simulink model "Traverse_system"  (R2022b)
settings: Solver=VariableStepAuto  StartTime=0.0  StopTime=30  RelTol=1e-3
undefined symbols (not defined in the file): C_pi_pod_trav_Ki, C_pi_pod_trav_Kp, C_pi_trav_gyro_simple, C_pi_trav_techo, gain_pod_trav, k_feed_gun_trav, k_feed_pod_trav, k_tgun_inv_plant, k_tpod_inv_plant, linear_feed_forward_GUN_trav_dist, linear_feed_forward_POD_trav_dist, linear_tgun_inv_plant, linear_tpod_inv_plant, trav_gyro_gain, trav_gyro_notch, trav_tacho_notch, trav_techo_plent_gain
libraries: slpidlib x4, simulink x1
settings Model: PacingRate=0.001000  Creator=ohadformanair  LastModifiedBy=ohadformanair
settings SolverCC: ZeroCrossAlgorithm=Adaptive
settings DataIOCC: SaveFormat=StructureWithTime
settings OptimizationCC: BlockReduction=off  OptimizeBlockIOStorage=off  BufferReuse=off
settings DebuggingCC: MaskedZcDiagnostic=none  IgnoredZcDiagnostic=none
settings ModelReferenceCC: EnableRefExpFcnMdlSchedulingChecks=on

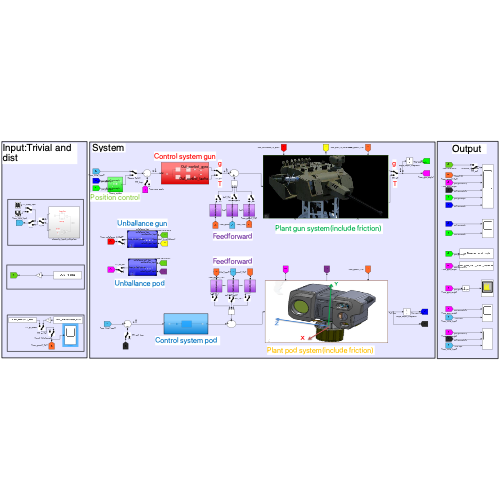
[thumbnail: Simulink's stored preview of the top-level diagram]
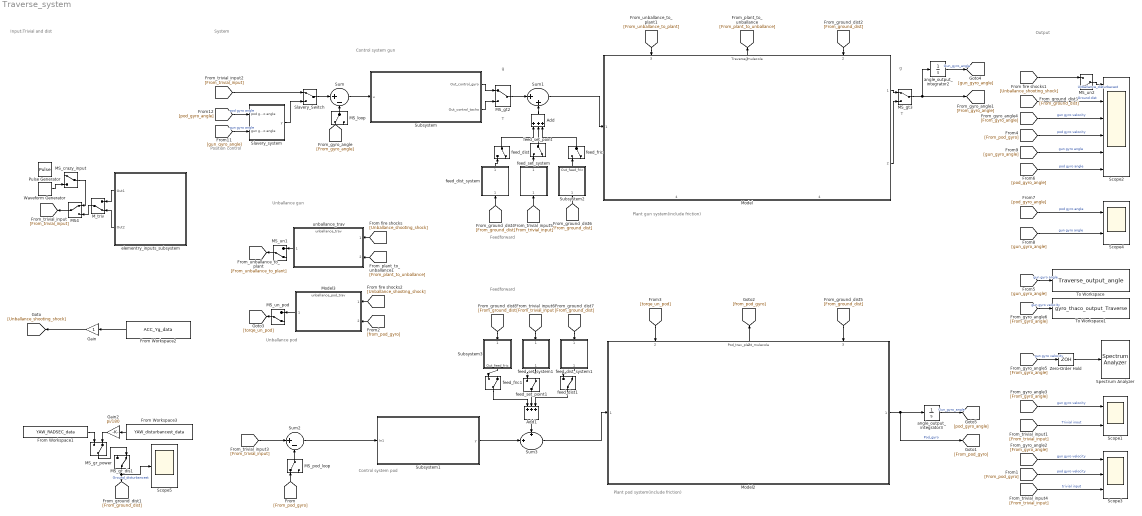
== system Traverse_system ==
  note: g
  note: g
  note: T
  note: T
  note: Plant gun system(include friction)
  note: Control system gun
  note: Unballance gun
  note: Input:Trivial and dist
  note: System
  note: Output
  note: Feedforward
  note: Plant pod system(include friction)
  note: Control system pod
  note: Unballance pod
  note: Position control
  note: Feedforward
  Add : Sum  Inputs=+++
  Add1 : Sum  Inputs=+++
  From Workspace1 : FromWorkspace  VariableName=YAW_RADSEC_data  SampleTime=-1
  From Workspace2 : FromWorkspace  VariableName=ACC_Yg_data  SampleTime=-1
  From Workspace3 : FromWorkspace  VariableName=YAW_disturbancest_data  SampleTime=-1
  Gain : Gain
  Gain2 : Gain  Gain=pi/180
  MS4 : ManualSwitch
  MS_crazy_input : ManualSwitch
  MS_gr_dis1 : ManualSwitch  CurrentSetting=0
  MS_gr_power : ManualSwitch  CurrentSetting=0
  MS_gt2 : ManualSwitch
  MS_gt3 : ManualSwitch
  MS_loop : ManualSwitch
  MS_pod_loop : ManualSwitch
  MS_un1 : ManualSwitch  CurrentSetting=0
  MS_un2 : ManualSwitch  CurrentSetting=0
  MS_un_pod : ManualSwitch  CurrentSetting=0
  M_triv : ManualSwitch  CurrentSetting=0
  Model : ModelReference  ModelNameDialog=Traverse_mulecola.slx  SimulationMode=Normal  ModelReferenceVersion=2.15
      settings: PortSchema="{\"entries\":[{\"content\":{\"sides\":[{\"content\":{\"connectorIds\":[\"In1\"]},\"type\":\"ConnectorPlacement.EquallySpacedRectSide\",\"uuid\":\"eac8caca-da38-417c-b045-6ec85fbd043e\"},{\"content\":{\"connectorIds\":[\"Out1\",\"Out2\"],\"side\":\"RIGHT\"},\"type\":\"ConnectorPlacement.EquallySpacedRectSide\",\"uuid\":\"64e84338-5cc1-4477-948e-9d784403bbd8\"},{\"content\":{\"connectorIds\":[\"In3\",\"Out3\",\"In2\"],\"side\":\"TOP\"},\"type\":\"ConnectorPlacement.EquallySpacedRectSide\",\"uuid\":\"1763b0b1-bf18-4a22-9773-91c6e4565572\"},{\"content\":{\"connectorIds\":[\"Out4\",\"In4\"],\"side\":\"BOTTOM\"},\"type\":\"ConnectorPlacement.EquallySpacedRectSide\",\"uuid\":\"ba992d88-ce65-42ad-a7d1-2242850eefcb\"}]},\"type\":\"ConnectorPlacement.EquallySpacedConnector\",\"uuid\":\"eba2f321-7b3d-4eb1-ab17-9114bc836124\"}],\"packageUris\":[\"http://schema.mathworks.com/mf0/Connector/R2020b\"],\"version\":\"1.0\"}"
      mask Display: image('/Users/ohadformanair/Desktop/צילום מסך 2022-12-07 ב-4.16.46.png'); % Use "Edit Image" on toolstrip to change.
  Model2 : ModelReference  ModelNameDialog=Pod_trav_plant_mulecola  SimulationMode=Normal  ModelReferenceVersion=1.15
      settings: PortSchema="{\"entries\":[{\"content\":{\"sides\":[{\"content\":{\"connectorIds\":[\"In1\"]},\"type\":\"ConnectorPlacement.EquallySpacedRectSide\",\"uuid\":\"257dd348-bb73-4a25-bb22-0aa44bc5c6b9\"},{\"content\":{\"connectorIds\":[\"Out1\"],\"side\":\"RIGHT\"},\"type\":\"ConnectorPlacement.EquallySpacedRectSide\",\"uuid\":\"83205adf-7330-4a40-93ca-0cec5d3c6531\"},{\"content\":{\"connectorIds\":[\"In2\",\"Out2\",\"In3\"],\"side\":\"TOP\"},\"type\":\"ConnectorPlacement.EquallySpacedRectSide\",\"uuid\":\"cb3612bd-e216-4a60-bf79-1bea0ce7796e\"}]},\"type\":\"ConnectorPlacement.EquallySpacedConnector\",\"uuid\":\"f84f5dbe-ed6b-457b-b8fc-4d1969f08882\"}],\"packageUris\":[\"http://schema.mathworks.com/mf0/Connector/R2020b\"],\"version\":\"1.0\"}"
      mask Display: image('/Users/ohadformanair/Desktop/צילום מסך 2022-12-07 ב-4.14.47.png'); % Use "Edit Image" on toolstrip to change.
  Model3 : ModelReference  ModelNameDialog=unballance_pod_trav.slx  SimulationMode=Normal  ModelReferenceVersion=1.12
  Pulse Generator : DiscretePulseGenerator  PulseType=Time based  Period=1  PulseWidth=50
  Scope1 : Scope  NumInputPorts=2
  Scope2 : Scope  NumInputPorts=6
  Scope3 : Scope  NumInputPorts=3
  Scope4 : Scope  NumInputPorts=2
  Scope5 : Scope
  Slavery_Switch : ManualSwitch
  Slavery_system : Subsystem
  Spectrum Analyzer : SpectrumAnalyzer
  Subsystem : Subsystem
  Subsystem1 : Subsystem  TreatAsAtomicUnit=on
  Subsystem2 : Subsystem
  Subsystem3 : Subsystem
  Sum : Sum  Inputs=|+-
  Sum1 : Sum  Inputs=|++
  Sum2 : Sum  Inputs=|+-
  Sum3 : Sum  Inputs=+|+||
  To Workspace : ToWorkspace  VariableName=Traverse_output_angle  SaveFormat=Timeseries  SampleTime=-1
  To Workspace1 : ToWorkspace  VariableName=gyro_thaco_output_Traverse  SaveFormat=Timeseries  SampleTime=-1
  Waveform Generator : simulink/Sources/Waveform Generator  OutMin=[]  OutMax=[]  OutDataTypeStr=double  SelectedSignal=1  Signals=sin(sawtooth(1,2,0),1,2)+Square(1,2,0,50)#Square(1,2,0,50)  BlockNames=MultiportSwitch_bb3116ca3c8c4cb#MultiportSwitch_6d83ebdfd0d2480  SampleTime=0.01
  Zero-Order Hold : ZeroOrderHold  SampleTime=0.001
  angle_output_integrator2 : Integrator
  angle_output_integrator3 : Integrator
  elementry_inputs_subsystem : Subsystem
  feed_dist : ManualSwitch  CurrentSetting=0
  feed_dist1 : ManualSwitch  CurrentSetting=0
  feed_dist_system : Subsystem
  feed_dist_system1 : Subsystem
  feed_fric : ManualSwitch  CurrentSetting=0
  feed_fric1 : ManualSwitch  CurrentSetting=0
  feed_set_point : ManualSwitch  CurrentSetting=0
  feed_set_point1 : ManualSwitch  CurrentSetting=0
  feed_set_system : Subsystem
  feed_set_system1 : Subsystem
  unballance_trav : ModelReference  ModelNameDialog=unballance_trav.slx  SimulationMode=Normal  ModelReferenceVersion=1.14
  wires:
  MS_loop/1 -> Sum/2
  MS_gt3/1 -> angle_output_integrator2/1, [From_gyro_angle]
  Model/1 -> MS_gt3/1
  Model/2 -> MS_gt3/2
  MS_gt2/1 -> Sum1/1
  MS_gr_power/1 -> MS_gr_dis1/2
  From Workspace3/1 -> Gain2/1
  Gain2/1 -> MS_gr_power/2
  Sum/1 -> Subsystem/1(u)
  Subsystem/1(Out_control_gyro) -> MS_gt2/1
  Subsystem/2(Out_control_tacho) -> MS_gt2/2
  elementry_inputs_subsystem/1(Out1) -> M_triv/1
  elementry_inputs_subsystem/2(Out2) -> M_triv/2
  From Workspace2/1 -> Gain/1
  unballance_trav/1 -> MS_un1/1
  From Workspace1/1 -> MS_gr_power/1
  Zero-Order Hold/1 -> Spectrum Analyzer/1
  MS_un2/1 -> Scope2/1  "Unballance_disturbacest"
  [From_gyro_angle] -> MS_loop/1
  MS_un1/1 -> [From_unballance_to_plant]
  [From_unballance_to_plant] -> Model/3
  [From_plant_to_unballance] -> unballance_trav/2
  Model/3 -> [From_plant_to_unballance]
  Gain/1 -> [Unballance_shooting_shock]
  [Unballance_shooting_shock] -> unballance_trav/1
  [Unballance_shooting_shock] -> MS_un2/1
  MS4/1 -> [From_trivial_input]
  [From_trivial_input] -> Slavery_Switch/1
  [From_trivial_input] -> Scope1/2  "Trivial inout"
  MS_gr_dis1/1 -> Scope5/1, [From_ground_dist]  "Ground_disturbancest"
  [From_ground_dist] -> Model/2
  [From_ground_dist] -> Scope2/2  "Ground dist"
  Add/1 -> Sum1/2
  feed_set_point/1 -> Add/2
  feed_dist/1 -> Add/1
  [From_ground_dist] -> feed_dist_system/1(feed_dist_input)
  feed_dist_system/1(feed_dist_output) -> feed_dist/1
  feed_set_system/1(feed_set_output) -> feed_set_point/1
  [From_trivial_input] -> feed_set_system/1(feed_set_input)
  Sum1/1 -> Model/1
  MS_crazy_input/1 -> MS4/1
  Waveform Generator/1 -> MS_crazy_input/2
  M_triv/1 -> MS4/2
  MS_pod_loop/1 -> Sum2/2
  [From_trivial_input] -> Sum2/1
  [From_trivial_input] -> Scope3/3  "trivial input"
  Model2/1 -> [From_pod_gyro], angle_output_integrator3/1  "Pod_gyro"
  Sum2/1 -> Subsystem1/1(In1)
  [From_ground_dist] -> Model2/3
  [From_pod_gyro] -> MS_pod_loop/1
  [From_pod_gyro] -> Scope3/2  "pod gyro velocity"
  Model2/2 -> [from_pod_gyro]
  [from_pod_gyro] -> Model3/2
  [Unballance_shooting_shock] -> Model3/1
  Model3/1 -> MS_un_pod/1
  MS_un_pod/1 -> [torqe_un_pod]
  [torqe_un_pod] -> Model2/2
  [From_pod_gyro] -> Scope2/4  "pod gyro velocity"
  Subsystem1/1(y) -> Sum3/2
  Sum3/1 -> Model2/1
  [From_gyro_angle] -> Scope3/1  "gun gyro velocity"
  [From_gyro_angle] -> Scope1/1  "gun gyro velocity"
  [From_gyro_angle] -> Zero-Order Hold/1  "gun gyro velocity"
  [From_gyro_angle] -> To Workspace1/1  "gun gyro velocity"
  angle_output_integrator2/1 -> [gun_gyro_angle]  "Gun_gyro_angle"
  [gun_gyro_angle] -> To Workspace/1  "gun gyro angle"
  angle_output_integrator3/1 -> [pod_gyro_angle]  "Gun_gyro_angle"
  [pod_gyro_angle] -> Scope4/1  "pod gyro angle"
  [pod_gyro_angle] -> Scope2/6  "pod gyro angle"
  [gun_gyro_angle] -> Scope4/2  "gun gyro angle"
  [gun_gyro_angle] -> Scope2/5  "gun gyro angle"
  [From_gyro_angle] -> Scope2/3  "gun gyro velocity"
  [From_ground_dist] -> Subsystem2/1(In_dist_velocity)
  feed_fric/1 -> Add/3
  Add1/1 -> Sum3/1
  Slavery_system/1(y) -> Slavery_Switch/2
  [gun_gyro_angle] -> Slavery_system/2(gun gyro angle)  "gun gyro angle"
  [pod_gyro_angle] -> Slavery_system/1(pod gyro angle)  "pod gyro angle"
  Slavery_Switch/1 -> Sum/1
  [From_ground_dist] -> feed_dist_system1/1(feed_dist_input)
  [From_ground_dist] -> Subsystem3/1(In_dist_velocity)
  feed_dist_system1/1(feed_dist_output) -> feed_dist1/1
  feed_set_system1/1(feed_set_output) -> feed_set_point1/1
  [From_trivial_input] -> feed_set_system1/1(feed_set_input)
  feed_set_point1/1 -> Add1/2
  feed_fric1/1 -> Add1/1
  feed_dist1/1 -> Add1/3
  Subsystem3/1(Out_feed_fric) -> feed_fric1/1
  Subsystem2/1(Out_feed_fric) -> feed_fric/1

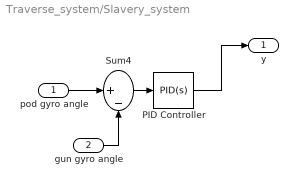
== system Traverse_system/Slavery_system ==
  pod gyro angle : Inport
  gun gyro angle : Inport  Port=2
  PID Controller : slpidlib/PID Controller  Controller=PID  Form=Parallel  TimeDomain=Continuous-time  UseExternalTs=off  SampleTime=-1  IntegratorMethod=Forward Euler  FilterMethod=Forward Euler  ControllerParametersSource=internal  P=37.221067348726+30  I=12.6865441571092  UseKiTs=off  D=0.178527594606658  N=4458.90311859589  UseFilter=on  TunerSelectOption=Transfer Function Based (PID Tuner App)  InitialConditionSource=internal  InitialConditionForIntegrator=0  InitialConditionForFilter=0  DifferentiatorICPrevScaledInput=0  ExternalReset=none  TrackingMode=off  Kt=1  LimitOutput=off  SatLimitsSource=internal  UpperSaturationLimit=inf  LowerSaturationLimit=-inf  LinearizeAsGain=on  AntiWindupMode=none  Kb=1  LimitIntegrator=off  UpperIntegratorSaturationLimit=inf  LowerIntegratorSaturationLimit=-inf  POutMin=[]  POutMax=[]  IOutMin=[]  IOutMax=[]  DOutMin=[]  DOutMax=[]  NOutMin=[]  NOutMax=[]  SumOutMin=[]  SumOutMax=[]  SaturationOutMin=[]  SaturationOutMax=[]  PParamMin=[]  PParamMax=[]  IParamMin=[]  IParamMax=[]  DParamMin=[]  DParamMax=[]  NParamMin=[]  NParamMax=[]  KbParamMin=[]  KbParamMax=[]  KtParamMin=[]  KtParamMax=[]  KbOutMin=[]  KbOutMax=[]  KtOutMin=[]  KtOutMax=[]  IntegratorOutMin=[]  IntegratorOutMax=[]  FilterOutMin=[]  FilterOutMax=[]  SumI1OutMin=[]  SumI1OutMax=[]  SumI2OutMin=[]  SumI2OutMax=[]  SumI3OutMin=[]  SumI3OutMax=[]  SumI4OutMin=[]  SumI4OutMax=[]  SumDOutMin=[]  SumDOutMax=[]  DifferentiatorOutMin=[]  DifferentiatorOutMax=[]  FilterDiffOutCoefMin=[]  FilterDiffOutCoefMax=[]  ReciprocalOutMin=[]  ReciprocalOutMax=[]  SumDenOutMin=[]  SumDenOutMax=[]  SumNumOutMin=[]  SumNumOutMax=[]  DivideOutMin=[]  DivideOutMax=[]  UdiffTsProdOutMin=[]  UdiffTsProdOutMax=[]  NTsProdOutMin=[]  NTsProdOutMax=[]  UintegralTsProdOutMin=[]  UintegralTsProdOutMax=[]  UngainTsProdOutMin=[]  UngainTsProdOutMax=[]  ClampingZeroOutDataTypeStr=Inherit: Inherit via back propagation  ClampingZeroOutMin=[]  ClampingZeroOutMax=[]  FilterDenConstantOutDataTypeStr=Inherit: Inherit via back propagation  FilterDenConstantOutMin=[]  FilterDenConstantOutMax=[]  PCopyOutDataTypeStr=Inherit: Inherit via back propagation  PCopyOutMin=[]  PCopyOutMax=[]  NCopyOutDataTypeStr=Inherit: Inherit via back propagation  NCopyOutMin=[]  NCopyOutMax=[]  IntegratorContinuousStateAttributes=''  IntegratorStateMustResolveToSignalObject=off  IntegratorRTWStateStorageClass=Auto  FilterContinuousStateAttributes=''  FilterStateMustResolveToSignalObject=off  FilterRTWStateStorageClass=Auto  ParallelPVariant=InternalParameters  IdealPVariant=Disabled  IVariant=InternalParameters  DVariant=InternalParameters  IntegratorVariant=Continuous  SatVariant=Disabled  AWVariant=Passthrough  PCopyVariant=Disabled  TRVariant=Disabled  FdbkBlocksVariant=Forward  IdealPFdbkVariant=Disabled  SatFdbkVariant=Disabled  DerivativeFilterVariant=ContFilter  NVariant=InternalParameters  NCopyVariant=Disabled  FilterICVariant=InternalICsFilter  IntegratorICVariant=InternalICs  ExternalResetVariant=Disabled  TRSumVariant=Passthrough  SumFdbkVariant=Disabled  SumVariant=Sum_PID  TsampFilterVariant=InternalTs  TsampNgainVariant=Passthrough  TsampIntegralVariant=Passthrough  ExternalSaturationOutDataTypeStr=Inherit: Same as second input
  Sum4 : Sum  Inputs=|+-
  y : Outport
  wires:
  pod gyro angle/1 -> Sum4/1
  PID Controller/1 -> y/1
  gun gyro angle/1 -> Sum4/2
  Sum4/1 -> PID Controller/1

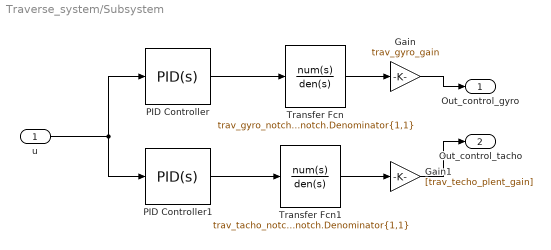
== system Traverse_system/Subsystem ==
  u : Inport
  Gain : Gain  Gain=trav_gyro_gain
  Gain1 : Gain  Gain=[trav_techo_plent_gain]
  PID Controller : slpidlib/PID Controller  Controller=PID  Form=Parallel  TimeDomain=Continuous-time  UseExternalTs=off  SampleTime=-1  IntegratorMethod=Forward Euler  FilterMethod=Forward Euler  ControllerParametersSource=internal  P=C_pi_trav_gyro_simple.Kp+1830  I=C_pi_trav_gyro_simple.Ki/0.9  UseKiTs=off  D=0  N=100  UseFilter=on  TunerSelectOption=Transfer Function Based (PID Tuner App)  InitialConditionSource=internal  InitialConditionForIntegrator=0  InitialConditionForFilter=0  DifferentiatorICPrevScaledInput=0  ExternalReset=none  TrackingMode=off  Kt=1  LimitOutput=off  SatLimitsSource=internal  UpperSaturationLimit=inf  LowerSaturationLimit=-inf  LinearizeAsGain=on  AntiWindupMode=none  Kb=1  LimitIntegrator=off  UpperIntegratorSaturationLimit=inf  LowerIntegratorSaturationLimit=-inf  POutMin=[]  POutMax=[]  IOutMin=[]  IOutMax=[]  DOutMin=[]  DOutMax=[]  NOutMin=[]  NOutMax=[]  SumOutMin=[]  SumOutMax=[]  SaturationOutMin=[]  SaturationOutMax=[]  PParamMin=[]  PParamMax=[]  IParamMin=[]  IParamMax=[]  DParamMin=[]  DParamMax=[]  NParamMin=[]  NParamMax=[]  KbParamMin=[]  KbParamMax=[]  KtParamMin=[]  KtParamMax=[]  KbOutMin=[]  KbOutMax=[]  KtOutMin=[]  KtOutMax=[]  IntegratorOutMin=[]  IntegratorOutMax=[]  FilterOutMin=[]  FilterOutMax=[]  SumI1OutMin=[]  SumI1OutMax=[]  SumI2OutMin=[]  SumI2OutMax=[]  SumI3OutMin=[]  SumI3OutMax=[]  SumI4OutMin=[]  SumI4OutMax=[]  SumDOutMin=[]  SumDOutMax=[]  DifferentiatorOutMin=[]  DifferentiatorOutMax=[]  FilterDiffOutCoefMin=[]  FilterDiffOutCoefMax=[]  ReciprocalOutMin=[]  ReciprocalOutMax=[]  SumDenOutMin=[]  SumDenOutMax=[]  SumNumOutMin=[]  SumNumOutMax=[]  DivideOutMin=[]  DivideOutMax=[]  UdiffTsProdOutMin=[]  UdiffTsProdOutMax=[]  NTsProdOutMin=[]  NTsProdOutMax=[]  UintegralTsProdOutMin=[]  UintegralTsProdOutMax=[]  UngainTsProdOutMin=[]  UngainTsProdOutMax=[]  ClampingZeroOutDataTypeStr=Inherit: Inherit via back propagation  ClampingZeroOutMin=[]  ClampingZeroOutMax=[]  FilterDenConstantOutDataTypeStr=Inherit: Inherit via back propagation  FilterDenConstantOutMin=[]  FilterDenConstantOutMax=[]  PCopyOutDataTypeStr=Inherit: Inherit via back propagation  PCopyOutMin=[]  PCopyOutMax=[]  NCopyOutDataTypeStr=Inherit: Inherit via back propagation  NCopyOutMin=[]  NCopyOutMax=[]  IntegratorContinuousStateAttributes=''  IntegratorStateMustResolveToSignalObject=off  IntegratorRTWStateStorageClass=Auto  FilterContinuousStateAttributes=''  FilterStateMustResolveToSignalObject=off  FilterRTWStateStorageClass=Auto  ParallelPVariant=InternalParameters  IdealPVariant=Disabled  IVariant=InternalParameters  DVariant=InternalParameters  IntegratorVariant=Continuous  SatVariant=Disabled  AWVariant=Passthrough  PCopyVariant=Disabled  TRVariant=Disabled  FdbkBlocksVariant=Forward  IdealPFdbkVariant=Disabled  SatFdbkVariant=Disabled  DerivativeFilterVariant=ContFilter  NVariant=InternalParameters  NCopyVariant=Disabled  FilterICVariant=InternalICsFilter  IntegratorICVariant=InternalICs  ExternalResetVariant=Disabled  TRSumVariant=Passthrough  SumFdbkVariant=Disabled  SumVariant=Sum_PID  TsampFilterVariant=InternalTs  TsampNgainVariant=Passthrough  TsampIntegralVariant=Passthrough  ExternalSaturationOutDataTypeStr=Inherit: Same as second input
  PID Controller1 : slpidlib/PID Controller  Controller=PID  Form=Parallel  TimeDomain=Continuous-time  UseExternalTs=off  SampleTime=-1  IntegratorMethod=Forward Euler  FilterMethod=Forward Euler  ControllerParametersSource=internal  P=C_pi_trav_techo.Kp  I=C_pi_trav_techo.Ki/20  UseKiTs=off  D=0  N=100  UseFilter=on  TunerSelectOption=Transfer Function Based (PID Tuner App)  InitialConditionSource=internal  InitialConditionForIntegrator=0  InitialConditionForFilter=0  DifferentiatorICPrevScaledInput=0  ExternalReset=none  TrackingMode=off  Kt=1  LimitOutput=off  SatLimitsSource=internal  UpperSaturationLimit=inf  LowerSaturationLimit=-inf  LinearizeAsGain=on  AntiWindupMode=none  Kb=1  LimitIntegrator=off  UpperIntegratorSaturationLimit=inf  LowerIntegratorSaturationLimit=-inf  POutMin=[]  POutMax=[]  IOutMin=[]  IOutMax=[]  DOutMin=[]  DOutMax=[]  NOutMin=[]  NOutMax=[]  SumOutMin=[]  SumOutMax=[]  SaturationOutMin=[]  SaturationOutMax=[]  PParamMin=[]  PParamMax=[]  IParamMin=[]  IParamMax=[]  DParamMin=[]  DParamMax=[]  NParamMin=[]  NParamMax=[]  KbParamMin=[]  KbParamMax=[]  KtParamMin=[]  KtParamMax=[]  KbOutMin=[]  KbOutMax=[]  KtOutMin=[]  KtOutMax=[]  IntegratorOutMin=[]  IntegratorOutMax=[]  FilterOutMin=[]  FilterOutMax=[]  SumI1OutMin=[]  SumI1OutMax=[]  SumI2OutMin=[]  SumI2OutMax=[]  SumI3OutMin=[]  SumI3OutMax=[]  SumI4OutMin=[]  SumI4OutMax=[]  SumDOutMin=[]  SumDOutMax=[]  DifferentiatorOutMin=[]  DifferentiatorOutMax=[]  FilterDiffOutCoefMin=[]  FilterDiffOutCoefMax=[]  ReciprocalOutMin=[]  ReciprocalOutMax=[]  SumDenOutMin=[]  SumDenOutMax=[]  SumNumOutMin=[]  SumNumOutMax=[]  DivideOutMin=[]  DivideOutMax=[]  UdiffTsProdOutMin=[]  UdiffTsProdOutMax=[]  NTsProdOutMin=[]  NTsProdOutMax=[]  UintegralTsProdOutMin=[]  UintegralTsProdOutMax=[]  UngainTsProdOutMin=[]  UngainTsProdOutMax=[]  ClampingZeroOutDataTypeStr=Inherit: Inherit via back propagation  ClampingZeroOutMin=[]  ClampingZeroOutMax=[]  FilterDenConstantOutDataTypeStr=Inherit: Inherit via back propagation  FilterDenConstantOutMin=[]  FilterDenConstantOutMax=[]  PCopyOutDataTypeStr=Inherit: Inherit via back propagation  PCopyOutMin=[]  PCopyOutMax=[]  NCopyOutDataTypeStr=Inherit: Inherit via back propagation  NCopyOutMin=[]  NCopyOutMax=[]  IntegratorContinuousStateAttributes=''  IntegratorStateMustResolveToSignalObject=off  IntegratorRTWStateStorageClass=Auto  FilterContinuousStateAttributes=''  FilterStateMustResolveToSignalObject=off  FilterRTWStateStorageClass=Auto  ParallelPVariant=InternalParameters  IdealPVariant=Disabled  IVariant=InternalParameters  DVariant=InternalParameters  IntegratorVariant=Continuous  SatVariant=Disabled  AWVariant=Passthrough  PCopyVariant=Disabled  TRVariant=Disabled  FdbkBlocksVariant=Forward  IdealPFdbkVariant=Disabled  SatFdbkVariant=Disabled  DerivativeFilterVariant=ContFilter  NVariant=InternalParameters  NCopyVariant=Disabled  FilterICVariant=InternalICsFilter  IntegratorICVariant=InternalICs  ExternalResetVariant=Disabled  TRSumVariant=Passthrough  SumFdbkVariant=Disabled  SumVariant=Sum_PID  TsampFilterVariant=InternalTs  TsampNgainVariant=Passthrough  TsampIntegralVariant=Passthrough  ExternalSaturationOutDataTypeStr=Inherit: Same as second input
  Transfer Fcn : TransferFcn  Numerator=trav_gyro_notch.Numerator{1,1}  Denominator=trav_gyro_notch.Denominator{1,1}
  Transfer Fcn1 : TransferFcn  Numerator=trav_tacho_notch.Numerator{1,1}  Denominator=trav_tacho_notch.Denominator{1,1}
  Out_control_gyro : Outport
  Out_control_tacho : Outport  Port=2
  wires:
  Gain1/1 -> Out_control_tacho/1
  Transfer Fcn/1 -> Gain/1
  u/1 -> PID Controller/1, PID Controller1/1
  PID Controller/1 -> Transfer Fcn/1
  Transfer Fcn1/1 -> Gain1/1
  Gain/1 -> Out_control_gyro/1
  PID Controller1/1 -> Transfer Fcn1/1

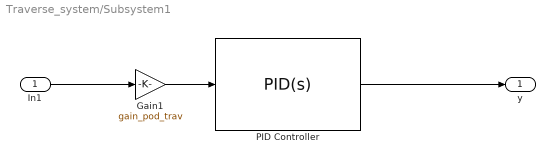
== system Traverse_system/Subsystem1 ==
  In1 : Inport
  Gain1 : Gain  Gain=gain_pod_trav
  PID Controller : slpidlib/PID Controller  Controller=PID  Form=Parallel  TimeDomain=Continuous-time  UseExternalTs=off  SampleTime=-1  IntegratorMethod=Forward Euler  FilterMethod=Forward Euler  ControllerParametersSource=internal  P=C_pi_pod_trav_Kp  I=C_pi_pod_trav_Ki  UseKiTs=off  D=0  N=100  UseFilter=on  TunerSelectOption=Transfer Function Based (PID Tuner App)  InitialConditionSource=internal  InitialConditionForIntegrator=0  InitialConditionForFilter=0  DifferentiatorICPrevScaledInput=0  ExternalReset=none  TrackingMode=off  Kt=1  LimitOutput=off  SatLimitsSource=internal  UpperSaturationLimit=inf  LowerSaturationLimit=-inf  LinearizeAsGain=on  AntiWindupMode=none  Kb=1  LimitIntegrator=off  UpperIntegratorSaturationLimit=inf  LowerIntegratorSaturationLimit=-inf  POutMin=[]  POutMax=[]  IOutMin=[]  IOutMax=[]  DOutMin=[]  DOutMax=[]  NOutMin=[]  NOutMax=[]  SumOutMin=[]  SumOutMax=[]  SaturationOutMin=[]  SaturationOutMax=[]  PParamMin=[]  PParamMax=[]  IParamMin=[]  IParamMax=[]  DParamMin=[]  DParamMax=[]  NParamMin=[]  NParamMax=[]  KbParamMin=[]  KbParamMax=[]  KtParamMin=[]  KtParamMax=[]  KbOutMin=[]  KbOutMax=[]  KtOutMin=[]  KtOutMax=[]  IntegratorOutMin=[]  IntegratorOutMax=[]  FilterOutMin=[]  FilterOutMax=[]  SumI1OutMin=[]  SumI1OutMax=[]  SumI2OutMin=[]  SumI2OutMax=[]  SumI3OutMin=[]  SumI3OutMax=[]  SumI4OutMin=[]  SumI4OutMax=[]  SumDOutMin=[]  SumDOutMax=[]  DifferentiatorOutMin=[]  DifferentiatorOutMax=[]  FilterDiffOutCoefMin=[]  FilterDiffOutCoefMax=[]  ReciprocalOutMin=[]  ReciprocalOutMax=[]  SumDenOutMin=[]  SumDenOutMax=[]  SumNumOutMin=[]  SumNumOutMax=[]  DivideOutMin=[]  DivideOutMax=[]  UdiffTsProdOutMin=[]  UdiffTsProdOutMax=[]  NTsProdOutMin=[]  NTsProdOutMax=[]  UintegralTsProdOutMin=[]  UintegralTsProdOutMax=[]  UngainTsProdOutMin=[]  UngainTsProdOutMax=[]  ClampingZeroOutDataTypeStr=Inherit: Inherit via back propagation  ClampingZeroOutMin=[]  ClampingZeroOutMax=[]  FilterDenConstantOutDataTypeStr=Inherit: Inherit via back propagation  FilterDenConstantOutMin=[]  FilterDenConstantOutMax=[]  PCopyOutDataTypeStr=Inherit: Inherit via back propagation  PCopyOutMin=[]  PCopyOutMax=[]  NCopyOutDataTypeStr=Inherit: Inherit via back propagation  NCopyOutMin=[]  NCopyOutMax=[]  IntegratorContinuousStateAttributes=''  IntegratorStateMustResolveToSignalObject=off  IntegratorRTWStateStorageClass=Auto  FilterContinuousStateAttributes=''  FilterStateMustResolveToSignalObject=off  FilterRTWStateStorageClass=Auto  ParallelPVariant=InternalParameters  IdealPVariant=Disabled  IVariant=InternalParameters  DVariant=InternalParameters  IntegratorVariant=Continuous  SatVariant=Disabled  AWVariant=Passthrough  PCopyVariant=Disabled  TRVariant=Disabled  FdbkBlocksVariant=Forward  IdealPFdbkVariant=Disabled  SatFdbkVariant=Disabled  DerivativeFilterVariant=ContFilter  NVariant=InternalParameters  NCopyVariant=Disabled  FilterICVariant=InternalICsFilter  IntegratorICVariant=InternalICs  ExternalResetVariant=Disabled  TRSumVariant=Passthrough  SumFdbkVariant=Disabled  SumVariant=Sum_PID  TsampFilterVariant=InternalTs  TsampNgainVariant=Passthrough  TsampIntegralVariant=Passthrough  ExternalSaturationOutDataTypeStr=Inherit: Same as second input
  y : Outport
  wires:
  In1/1 -> Gain1/1
  PID Controller/1 -> y/1
  Gain1/1 -> PID Controller/1

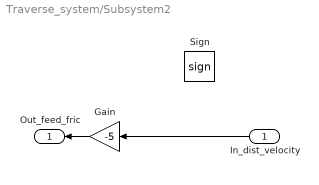
== system Traverse_system/Subsystem2 ==
  In_dist_velocity : Inport
  Gain : Gain  Gain=-5
  Sign : Signum
  Out_feed_fric : Outport
  wires:
  Gain/1 -> Out_feed_fric/1
  In_dist_velocity/1 -> Gain/1

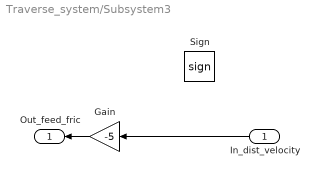
== system Traverse_system/Subsystem3 ==
  In_dist_velocity : Inport
  Gain : Gain  Gain=-5
  Sign : Signum
  Out_feed_fric : Outport
  wires:
  Gain/1 -> Out_feed_fric/1
  In_dist_velocity/1 -> Gain/1

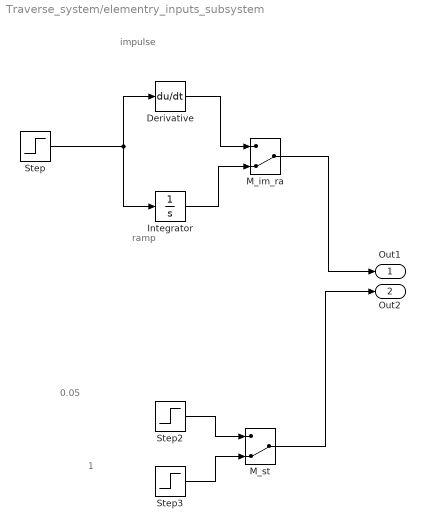
== system Traverse_system/elementry_inputs_subsystem ==
  note: 0.05
  note: 1
  note: ramp
  note: impulse
  Derivative : Derivative
  Integrator : Integrator
  M_im_ra : ManualSwitch  CurrentSetting=0
  M_st : ManualSwitch  CurrentSetting=0
  Step : Step  SampleTime=0
  Step2 : Step  After=0.05  SampleTime=0
  Step3 : Step  SampleTime=0
  Out1 : Outport
  Out2 : Outport  Port=2
  wires:
  Step/1 -> Integrator/1, Derivative/1
  M_im_ra/1 -> Out1/1
  Integrator/1 -> M_im_ra/2
  Step3/1 -> M_st/2
  Derivative/1 -> M_im_ra/1
  M_st/1 -> Out2/1
  Step2/1 -> M_st/1

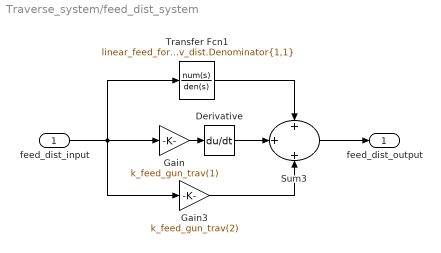
== system Traverse_system/feed_dist_system ==
  feed_dist_input : Inport
  Derivative : Derivative
  Gain : Gain  Gain=k_feed_gun_trav(1)
  Gain3 : Gain  Gain=k_feed_gun_trav(2)
  Sum3 : Sum  Inputs=+|+|+
  Transfer Fcn1 : TransferFcn  Numerator=linear_feed_forward_GUN_trav_dist.Numerator{1,1}  Denominator=linear_feed_forward_GUN_trav_dist.Denominator{1,1}
  feed_dist_output : Outport
  wires:
  Sum3/1 -> feed_dist_output/1
  Derivative/1 -> Sum3/2
  feed_dist_input/1 -> Gain/1, Gain3/1, Transfer Fcn1/1
  Transfer Fcn1/1 -> Sum3/1
  Gain/1 -> Derivative/1
  Gain3/1 -> Sum3/3

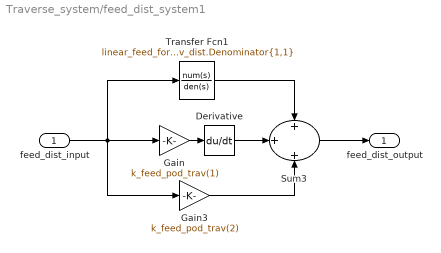
== system Traverse_system/feed_dist_system1 ==
  feed_dist_input : Inport
  Derivative : Derivative
  Gain : Gain  Gain=k_feed_pod_trav(1)
  Gain3 : Gain  Gain=k_feed_pod_trav(2)
  Sum3 : Sum  Inputs=+|+|+
  Transfer Fcn1 : TransferFcn  Numerator=linear_feed_forward_POD_trav_dist.Numerator{1,1}  Denominator=linear_feed_forward_POD_trav_dist.Denominator{1,1}
  feed_dist_output : Outport
  wires:
  Sum3/1 -> feed_dist_output/1
  Derivative/1 -> Sum3/2
  feed_dist_input/1 -> Gain/1, Gain3/1, Transfer Fcn1/1
  Transfer Fcn1/1 -> Sum3/1
  Gain/1 -> Derivative/1
  Gain3/1 -> Sum3/3

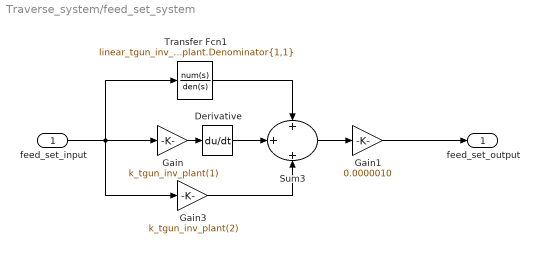
== system Traverse_system/feed_set_system ==
  feed_set_input : Inport
  Derivative : Derivative
  Gain : Gain  Gain=k_tgun_inv_plant(1)
  Gain1 : Gain  Gain=0.0000010
  Gain3 : Gain  Gain=k_tgun_inv_plant(2)
  Sum3 : Sum  Inputs=+|+|+
  Transfer Fcn1 : TransferFcn  Numerator=linear_tgun_inv_plant.Numerator{1,1}  Denominator=linear_tgun_inv_plant.Denominator{1,1}
  feed_set_output : Outport
  wires:
  Derivative/1 -> Sum3/2
  feed_set_input/1 -> Gain/1, Gain3/1, Transfer Fcn1/1
  Transfer Fcn1/1 -> Sum3/1
  Gain/1 -> Derivative/1
  Gain3/1 -> Sum3/3
  Sum3/1 -> Gain1/1
  Gain1/1 -> feed_set_output/1

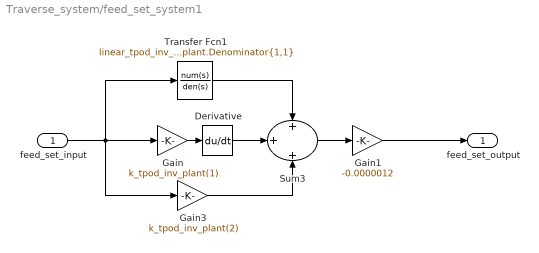
== system Traverse_system/feed_set_system1 ==
  feed_set_input : Inport
  Derivative : Derivative
  Gain : Gain  Gain=k_tpod_inv_plant(1)
  Gain1 : Gain  Gain=-0.0000012
  Gain3 : Gain  Gain=k_tpod_inv_plant(2)
  Sum3 : Sum  Inputs=+|+|+
  Transfer Fcn1 : TransferFcn  Numerator=linear_tpod_inv_plant.Numerator{1,1}  Denominator=linear_tpod_inv_plant.Denominator{1,1}
  feed_set_output : Outport
  wires:
  Derivative/1 -> Sum3/2
  feed_set_input/1 -> Gain/1, Gain3/1, Transfer Fcn1/1
  Transfer Fcn1/1 -> Sum3/1
  Gain/1 -> Derivative/1
  Gain3/1 -> Sum3/3
  Sum3/1 -> Gain1/1
  Gain1/1 -> feed_set_output/1
